simulink model "hiv_model_ekf_template"  (R2021a)
settings: Solver=VariableStepAuto  StartTime=0.0  StopTime=10.0  RelTol=1e-3
values from neighbouring files (symbols this model uses):
  Delta = 0.01    [init.m]
  Theta = [0.25 50 0.25 10 0.01 0.0045]'    [init.m]
  xdash0 = [1000 550 0.0001]'    [init.m]
  xdash12RL = [1000 550]'    [init.m]
settings Model: Creator=schauer  LastModifiedBy=Tomo
settings SolverCC: AlgebraicLoopSolver=TrustRegion
settings DebuggingCC: SFMachineParentedDataDiag=warning

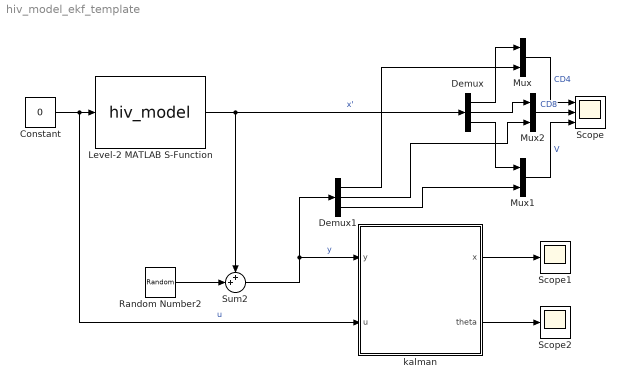
== system hiv_model_ekf_template ==
  Constant : Constant  Value=0
  Demux : Demux  Outputs=3
  Demux1 : Demux  Outputs=3
  Level-2 MATLAB S-Function : M-S-Function  FunctionName=hiv_model  Parameters=xdash0,Theta,xdash12RL
  Mux : Mux  Inputs=2
  Mux1 : Mux  Inputs=2
  Mux2 : Mux  Inputs=2
  Random Number2 : RandomNumber  Variance=[100 100 10^-5]  SampleTime=Delta
  Scope : Scope  NumInputPorts=3
  Scope1 : Scope
  Scope2 : Scope
  Sum2 : Sum  Inputs=++|
  kalman : MATLAB Function  TreatAsAtomicUnit=on
  wires:
  Constant/1 -> kalman/2(u), Level-2 MATLAB S-Function/1  "u"
  Level-2 MATLAB S-Function/1 -> Demux/1, Sum2/1  "x'"
  Mux/1 -> Scope/1  "CD4"
  Demux/1 -> Mux/1
  Demux/3 -> Mux1/1
  Mux1/1 -> Scope/3  "V"
  Sum2/1 -> kalman/1(y), Demux1/1  "y"
  Random Number2/1 -> Sum2/2
  Mux2/1 -> Scope/2  "CD8"
  Demux/2 -> Mux2/1
  Demux1/1 -> Mux/2
  Demux1/2 -> Mux2/2
  Demux1/3 -> Mux1/2
  kalman/1(x) -> Scope1/1
  kalman/2(theta) -> Scope2/1

== matlab function hiv_model_ekf_template/kalman ==
  settings: updateMethod=DISCRETE
  data: y input; u input; x output; theta output
function [x, theta]  = fcn(y, u)

% init
persistent x_k P
if isempty(x_k)
    x_0 = [1000 550 0.0001]';
    th_wahr = [0.25 50 0.25 10 0.01 0.0045]';
    th_0 = th_wahr * (1+0.3);
    P = 1.3^2 * eye(9, 9);
    x_k = zeros(1, 9);
    x_k(1:3) = x_0;
    x_k(4:9) = th_0;
end

Delta = 0.01;
x_RL = [1000 550]';
noise = -1 + 2*rand(3, 1);
noise = [100 100 10e-5]' .* noise;
Z = eye(3);
Z(1,1) = noise(1); Z(2,2) = noise(2); Z(3,3) = noise(3);

A_k = [(1-Delta*(x_k(4)-x_k(5)*x_k(3))),0,-Delta*x_k(4)*x_k(1),...
     Delta*(x_RL(1)-x_k(1)),Delta*x_k(1)*x_k(3),0,0,0,0;...                       
     0,(1-Delta*(x_k(6)+x_k(7)*x_k(3))),Delta*x_k(7)*x_k(2),0,0,...
     Delta*(x_RL(2)-x_k(2)),Delta*x_k(2)*x_k(3),0,0;...                           
     Delta*x_k(8)*x_k(3),-Delta*x_k(9)*x_k(3),1+Delta*(x_k(8)*x_k(1)-...
     x_k(9)*x_k(2)),0,0,0,0,Delta*x_k(1)*x_k(3),-Delta*x_k(2)*x_k(3);...    
     zeros(1,3),1,zeros(1,5);...                                            
     zeros(1,4),1,zeros(1,4);...                                            
     zeros(1,5),1,zeros(1,3);...                                            
     zeros(1,6),1,zeros(1,2);...                                            
     zeros(1,7),1,0;...                                                     
     zeros(1,8),1]; 

C = eye(3, 9);

% Prediktion
x_k = [x_k(1)+Delta*(x_k(4)*(x_RL(1)-x_k(1))-x_k(5)*x_k(1)*x_k(3))+Z(1),...
      x_k(2)+Delta*(x_k(6)*(x_RL(2)-x_k(2))+x_k(7)*x_k(2)*x_k(3))+Z(2),...
      x_k(3)+Delta*(x_k(3)*(x_k(8)*x_k(1)-x_k(9)*x_k(2))-u)+Z(3),...
      x_k(4:9)];
P = A_k*P*A_k';

% Update
C_k1 = C;
K = P*C_k1' * (Z + C_k1*P*C_k1')^-1;
h_k = x_k(1:3);
x_k = x_k + (K*(y - h_k'))'; % x_k1
P = P - K*C_k1*P; % P_k1

% output
x = x_k(1:3);
theta = x_k(4:9);
